simulink model "ModelEnv_Test_RL_4"  (R2020b)
settings: Solver=VariableStepAuto  StartTime=0.0  StopTime=24  RelTol=1e-3
values from neighbouring files (symbols this model uses):
  alpha = 0.15    [AgentSaboteur.m]    (also in Test1_code.m; TesterUnAgent.m; test_RL_code.m; test_RL_code_v2.m)
  Atz = -0.15    [AgentSaboteur.m]    (also in Test1_code.m; TesterUnAgent.m; test_RL_code.m; test_RL_code_v2.m)
  Bd = 0.03    [AgentSaboteur.m]    (also in Test1_code.m; TesterUnAgent.m; test_RL_code.m; test_RL_code_v2.m)
  Bh = mdot/(3*M)    (= 0.164794600011)    [AgentSaboteur.m]    (also in Test1_code.m; TesterUnAgent.m; test_RL_code.m; test_RL_code_v2.m)
  gama = 0.7    [AgentSaboteur.m]    (also in Test1_code.m; TesterUnAgent.m; test_RL_code.m; test_RL_code_v2.m)
  theta = 0.15    [AgentSaboteur.m]    (also in Test1_code.m; TesterUnAgent.m; test_RL_code.m; test_RL_code_v2.m)
  Ts = 0.2    [AgentSaboteur.m]    (also in Test1_code.m = 1; TesterUnAgent.m; testBlanc.m = 0.1; test_RL_code.m = 0.4)
  Tz_init = Tout(1)    [AgentSaboteur.m]    (also in Test1_code.m; TesterUnAgent.m; testBlanc.m; test_RL_code.m)
libraries: dspsrcs4 x2, rllib x1
settings Model: Creator=masdoua1  LastModifiedBy=masdoua1

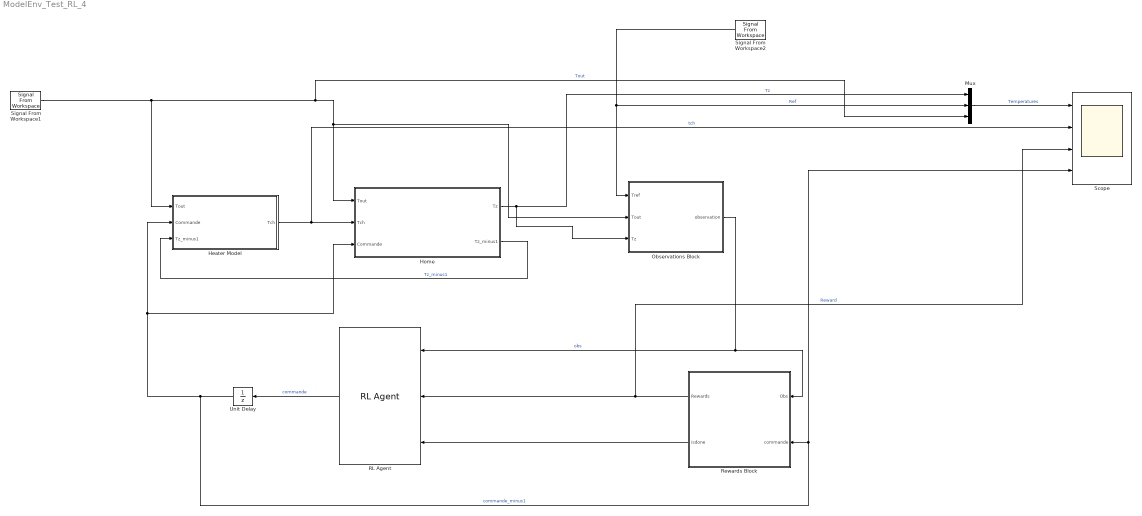
== system ModelEnv_Test_RL_4 ==
  Heater Model : Subsystem
  Home : Subsystem
  Mux : Mux  Inputs=3
  Observations Block : Subsystem
  RL Agent : rllib/RL Agent  Agent=agent  ProvideReward=on  ProvideIsDone=on  ProvideCumRwd=off  TreatAsDirectFeedthrough=on  CollectLoggedSignals=on  CollectModelStates=on
  Rewards Block : Subsystem
  Scope : Scope  NumInputPorts=4
  Signal From Workspace1 : dspsrcs4/Signal From Workspace  X=Tout  Ts=1  nsamps=1  OutputAfterFinalValue=Setting to zero  ignoreOrWarnInputAndFrameLengths=off  OutputFrames=off
  Signal From Workspace2 : dspsrcs4/Signal From Workspace  X=Ref  Ts=1  nsamps=1  OutputAfterFinalValue=Setting to zero  ignoreOrWarnInputAndFrameLengths=off  OutputFrames=off
  Unit Delay : UnitDelay  SampleTime=-1  HasFrameUpgradeWarning=on
  wires:
  Observations Block/1(observation) -> Rewards Block/1(Obs), RL Agent/1  "obs"
  Heater Model/1(Tch) -> Scope/2, Home/2(Tch)  "tch"
  Rewards Block/1(Rewards) -> Scope/3, RL Agent/2  "Reward"
  Unit Delay/1 -> Rewards Block/2(commande), Scope/4, Heater Model/2(Commande), Home/3(Commande)  "commande_minus1"
  Home/1(Tz) -> Observations Block/3(Tz), Mux/1  "Tz"
  Signal From Workspace2/1 -> Mux/2, Observations Block/1(Tref)  "Ref"
  Mux/1 -> Scope/1  "Temperatures"
  Home/2(Tz_minus1) -> Heater Model/3(Tz_minus1)  "Tz_minus1"
  Rewards Block/2(isdone) -> RL Agent/3
  Signal From Workspace1/1 -> Heater Model/1(Tout), Observations Block/2(Tout), Home/1(Tout), Mux/3  "Tout"
  RL Agent/1 -> Unit Delay/1  "commande"

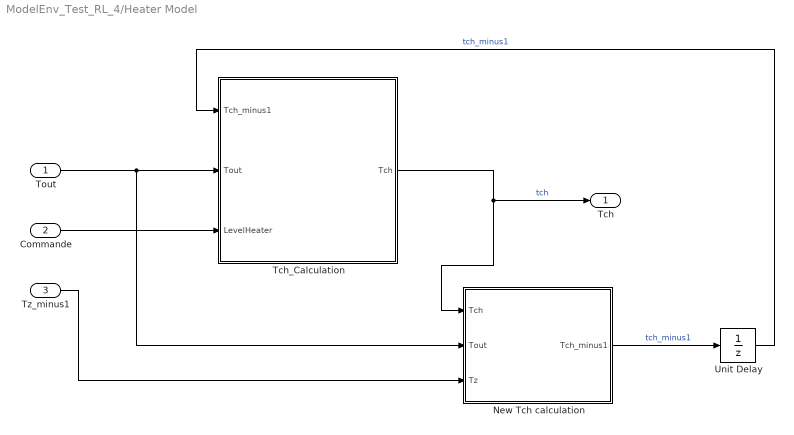
== system ModelEnv_Test_RL_4/Heater Model ==
  Tout : Inport
  Commande : Inport  Port=2
  Tz_minus1 : Inport  Port=3
  New Tch calculation : Subsystem
  Tch_Calculation : MATLAB Function  TreatAsAtomicUnit=on
  Unit Delay : UnitDelay  SampleTime=-1  HasFrameUpgradeWarning=on
  Tch : Outport
  wires:
  Tout/1 -> New Tch calculation/2(Tout), Tch_Calculation/2(Tout)
  Commande/1 -> Tch_Calculation/3(LevelHeater)
  Tch_Calculation/1(Tch) -> New Tch calculation/1(Tch), Tch/1  "tch"
  Unit Delay/1 -> Tch_Calculation/1(Tch_minus1)  "tch_minus1"
  Tz_minus1/1 -> New Tch calculation/3(Tz)
  New Tch calculation/1(Tch_minus1) -> Unit Delay/1  "tch_minus1"

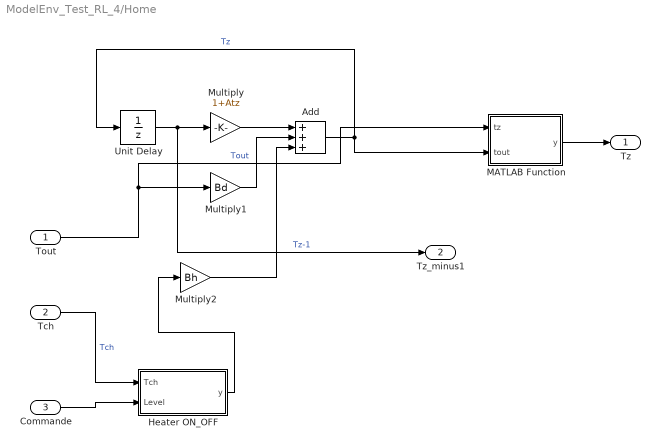
== system ModelEnv_Test_RL_4/Home ==
  Tout : Inport
  Tch : Inport  Port=2
  Commande : Inport  Port=3
  Add : Sum  Inputs=+++
  Heater ON_OFF : MATLAB Function  TreatAsAtomicUnit=on
  MATLAB Function : MATLAB Function  TreatAsAtomicUnit=on
  Multiply : Gain  Gain=1+Atz
  Multiply1 : Gain  Gain=Bd
  Multiply2 : Gain  Gain=Bh
  Unit Delay : UnitDelay  InitialCondition=Tz_init  SampleTime=Ts  HasFrameUpgradeWarning=on
  Tz : Outport
  Tz_minus1 : Outport  Port=2
  wires:
  Multiply/1 -> Add/1
  Unit Delay/1 -> Tz_minus1/1, Multiply/1  "Tz-1"
  Tout/1 -> MATLAB Function/1(tz), Multiply1/1  "Tout"
  Multiply1/1 -> Add/2
  Add/1 -> Unit Delay/1, MATLAB Function/2(tout)  "Tz"
  Multiply2/1 -> Add/3
  Commande/1 -> Heater ON_OFF/2(Level)
  Tch/1 -> Heater ON_OFF/1(Tch)  "Tch"
  Heater ON_OFF/1(y) -> Multiply2/1
  MATLAB Function/1(y) -> Tz/1

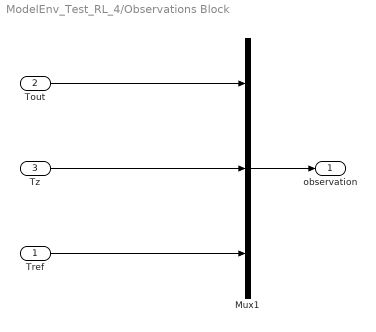
== system ModelEnv_Test_RL_4/Observations Block ==
  Tref : Inport
  Tout : Inport  Port=2
  Tz : Inport  Port=3
  Mux1 : Mux  Inputs=3
  observation : Outport
  wires:
  Mux1/1 -> observation/1
  Tz/1 -> Mux1/2
  Tout/1 -> Mux1/1
  Tref/1 -> Mux1/3

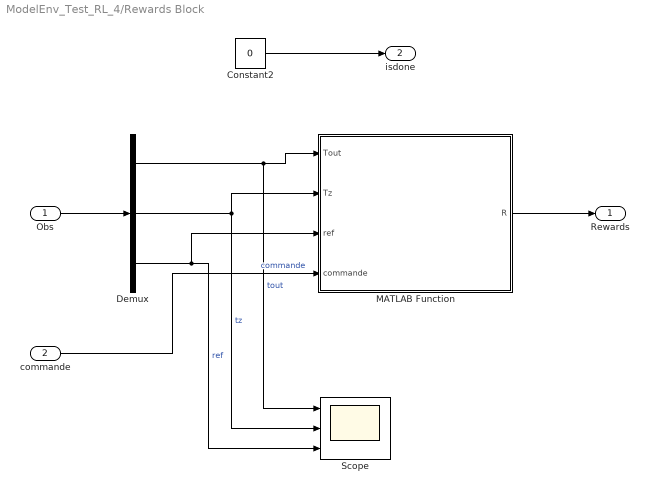
== system ModelEnv_Test_RL_4/Rewards Block ==
  Obs : Inport
  commande : Inport  Port=2
  Constant2 : Constant  Value=0
  Demux : Demux  Outputs=3
  MATLAB Function : MATLAB Function  TreatAsAtomicUnit=on
  Scope : Scope  NumInputPorts=3
  Rewards : Outport  VectorParamsAs1DForOutWhenUnconnected=off
  isdone : Outport  Port=2  VectorParamsAs1DForOutWhenUnconnected=off
  wires:
  Constant2/1 -> isdone/1
  MATLAB Function/1(R) -> Rewards/1
  Obs/1 -> Demux/1
  Demux/1 -> Scope/1, MATLAB Function/1(Tout)  "tout"
  Demux/2 -> MATLAB Function/2(Tz), Scope/2  "tz"
  Demux/3 -> MATLAB Function/3(ref), Scope/3  "ref"
  commande/1 -> MATLAB Function/4(commande)  "commande"

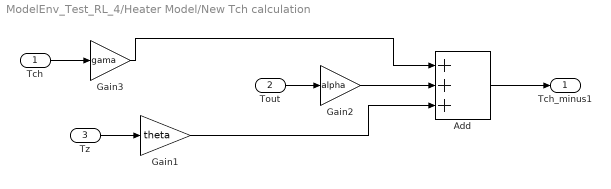
== system ModelEnv_Test_RL_4/Heater Model/New Tch calculation ==
  Tch : Inport
  Tout : Inport  Port=2
  Tz : Inport  Port=3
  Add : Sum  Inputs=+++
  Gain1 : Gain  Gain=theta
  Gain2 : Gain  Gain=alpha
  Gain3 : Gain  Gain=gama
  Tch_minus1 : Outport
  wires:
  Add/1 -> Tch_minus1/1
  Gain1/1 -> Add/3
  Tz/1 -> Gain1/1
  Tout/1 -> Gain2/1
  Gain2/1 -> Add/2
  Tch/1 -> Gain3/1
  Gain3/1 -> Add/1

== matlab function ModelEnv_Test_RL_4/Heater Model/Tch_Calculation ==
  data: Tch_minus1 input; Tout input; LevelHeater input; Tch output
function Tch = fcn(Tch_minus1, Tout, LevelHeater)
    
    if Tout > Tch_minus1
        Tch_minus1 = Tout+0.2; 
    end
    
    Tch = Tch_minus1 + LevelHeater;

== matlab function ModelEnv_Test_RL_4/Rewards Block/MATLAB Function ==
  data: Tout input; R output; Tz input; ref input; commande input
function R = fcn(Tout,Tz, ref, commande)

R1 = 0; R2 = 0; R3 = 0;

err = abs(ref - Tz);

% if err <= 0.1
%     R1 = 100;
% elseif err <= 2
%     R1 = 50;
% elseif err <= 4
%     R1 = 10;
% elseif err <= 6
%     R1 = -10;
% else
%     R1 = -100;
% end

% err = abs(Tz-ref);

% if err == 0
%     R1 = 100;
% else
%     R1 = 10*(1/err);
% end

% R1 = - 100 * err;

%% Regulation => erreur = 0.
R1 = -1 * err;

if (err < 1)
    R2 = 10;
end
%% Minimisation energie => Minimisation (Commande)
% R2 = -10 * commande;

R = R1 + R2 + R3;

== matlab function ModelEnv_Test_RL_4/Home/Heater ON_OFF ==
  data: Tch input; Level input; y output
function y = fcn(Tch, Level)
y = Tch;
if Level ==0
        y = 0;
end

== matlab function ModelEnv_Test_RL_4/Home/MATLAB Function ==
  data: tz input; tout input; y output
function y = fcn(tz, tout)
y = tz;
    if tz < tout
        y = tout;
    end
